simulink library "libbha_kinematic"  (R2015b)
settings: Solver=FixedStepDiscrete  StartTime=0.0  StopTime=Inf  FixedStep=0.004  RelTol=1e-3
PostLoadFcn:
  | , if any(exist('dsrtsu_mdlpostloadfcn', 'file') == [2, 3, 6]), try dsrtsu_mdlpostloadfcn('Execute', bdroot); catch fprintf('Error in PostLoadFcn (dsrtsu_mdlpostloadfcn) for model "%s":\n %s\n', bdroot, lasterr); end, end,
undefined symbols (not defined in the file or in its folder): BHA, BHASIM
libraries: libbha_kinematic x14
(part 3 of 3)

== matlab function libbha_kinematic/BHA_Kin_DirDiff_2ndO_CC_cont/J_general & J_specific ==
  data: h output; k output; q input; dot_q input; H_1b_w input; J_allg_kK output; r_i input; h_ih input; h_ib input; J_spez_kK_kA output; dot_J_allg_kK output; dot_J_spez_kK_kA output
function [h, k, J_allg_kK, J_spez_kK_kA, dot_J_allg_kK, dot_J_spez_kK_kA]   = Jacobi_CC_continuum(q, dot_q, H_1b_w, r_i, h_ih, h_ib)
n = 3;
% XXXXXXXXXXXXXXXXXXXXXXXXXXXXXXXXXXXXXXXXXXXXXXXXXXXXXXXXXXXXXXXXXXXXXXXXX
% Analytische Berechnung der Jacobi-Matrizen J_general und J_specific 
% - Modell - Constant Curvature Continuum
%
% Ansatz:
% h     = f_general(k)
% k     = f_specific(q)
% ==>
% h     = f_general(f_specific(q))
%
% J_general     = dh / dk
% J_specific    = dk / dq
%
% mit:
% q     = [ell_11, ell_12, ell_13, ell_21, ell_22, ell_23, ell_31, ell_32, ell_33]
% k     = [phi_1, kappa_1, ell_1, phi_2, kappa_2, ell_2, phi_3, kappa_3, ell_3]
% h     = [ H_1,1,  H_2,1,  H_3,1,  H_1,2,  H_2,2,  H_3,2,  H_1,3,  H_2,3,  H_3,3,  H_1,4,  H_2,4,  H_3,4]
%           1       2       3       4       5       6       7       8       9       10      11      12   
%
% Input:
%   q           [3nx1]  Zustandsvektor der Gelenkkoordinaten (Bogenlänge der Aktoren)
%   H_1b_w   [4x4]   Homogene Transformation: Koordinatensystem 1b
%                       relativ zum Weltsystem
%
% Output:
%   h           [12x1]  Pose des TCP (Homohene Transformation in Vektor geschrieben, ohne Zeile 0,0,0,1)
%   J_general   [12x3n] Allgemeingültige Jacobi-Matrix für kontinuierliche Manipulatoren
%   k           [3nx1]  Konfigurationszustand
%   J_specific  [3nx3n] Manipulator-spezifische Jacobimatrix (3-Aktuator Kontinuum Manipulator)
%
% Parameter:
%   n           [1x1]   Anzahl der Sektionen
%   r_i         [1xn]   Radialer Abstand der Aktoren pro Sektion
%   h_ib        [1xn]   Höhe der Sektionsbasis pro Sektion
%   h_ih        [1xn]   Höhe des Sektionskopfs pro Sektion
%
% Stand: 21.01.2013     Tobias Mahl
% XXXXXXXXXXXXXXXXXXXXXXXXXXXXXXXXXXXXXXXXXXXXXXXXXXXXXXXXXXXXXXXXXXXXXXXXX
    
    eps_kappa_i = 1e-7*ones(1, n);
    eps_wurzel_i= 1e-6*ones(1, n);% Berechnen!
    
    % Direkte Kinematik
    k = f_spez_kK_kA(n, q, r_i);
    [H_nh_w, H_ih_ib] = f_allg_kK(n, k, h_ib, h_ih, H_1b_w, eps_kappa_i);
    h = H2h(H_nh_w);
    
    % Direkte differentielle Kinematik 1. Ordnung
    J_spez_kK_kA = df_spez_kK_kA_dq(n, q, r_i, k, eps_wurzel_i);
    [J_allg_kK, dh_Ih_Ib_dk_I_all] = df_allg_kK_dk(n, k, h_ib, h_ih, H_1b_w, H_ih_ib, eps_kappa_i);
    
    % Direkte differentielle Kinematik 2. Ordnung
    dot_J_spez_kK_kA = dot_dk_dq(n, q, dot_q, r_i);
    
    ddH_nh_w_dk_dk = clc_ddH_nh_w_dk_dk(n, k, H_1b_w, H_ih_ib, dh_Ih_Ib_dk_I_all, h_ib, h_ih);
    dot_k = J_spez_kK_kA * dot_q;
    dot_J_allg_kK = ddf_allg_kK_dk_dt(n, dot_k, ddH_nh_w_dk_dk);
end

%% XXXXXXXXXXXXXXXXXXXXXXXXXXXXXX Allgemeines XXXXXXXXXXXXXXXXXXXXXXXXXXXXX

function h = H2h(H)
% Transformation:
%   homogene Transformation H --> vektorielle Repräsentation h
%                     H {4x4} --> h {12x1}

    h = reshape(H(1:3,:), [12,1]);
end

function H = h2H(h)
% Transformation:
%   vektorielle Repräsentation h --> homogene Transformation H
%                       h {12x1} --> H {4x4}

    H = [reshape(h, [3,4]); 0,0,0,1];
end

%% XXXXXXXXXXXXXXXXXXXXXXXXXXXXXX f_spez XXXXXXXXXXXXXXXXXXXXXXXXXXXXXXXXXX
function k = f_spez_kK_kA(n, q, r_i)
% Berechnung der Transformation
% Aktorbogenlängen q --> Konfigurationszustand k  
% des kontinuierlichen Roboters gemäß der Abbildung:
% k = f_specific(q)
% 
% Input:
%   q  [3nx1]   Aktorbogenlängen (kontinuierlich biegender Aktor)
%
% Output:
%   k     [3nx1]   Konfigurationszustand mit (phi_i, kappa_i, ell_i)
%
% Parameter:
%   r_i     [1xn]   Radiale Abständ der Aktoren je Sektion i
    
    k = zeros(3*n, 1);
    for ii=1:n
        k((1:3)+(ii-1)*3, 1) = f_spez_kK_kA_I(q((1:3)+(ii-1)*3, 1), r_i(ii));
    end
end

function k_I = f_spez_kK_kA_I(q_I, r_I)
% Berechnung der Transformation
% Aktorbogenlängen q_I --> Konfigurationszustand [phi_I, kappa_I, ell_I]  
% einer einzelnen Sektion gemäß der Abbildung:
% k_I = f_specific_I(q_I)
% 
% Input:
%   q_I  [3x1]   Aktorbogenlängen (kontinuierlich biegender Aktor)
%
% Output:
%   k_I     [3x1]   Konfigurationszustand (phi_I, kappa_I, ell_I)
%
% Parameter:
%   r_I     [1x1]   Radialer Abstand der Aktoren

    wurzel = sqrt(max([0, q_I(1,1)^2 + q_I(2,1)^2 + q_I(3,1)^2 - q_I(1,1)*q_I(2,1) - q_I(1,1)*q_I(3,1) - q_I(2,1)*q_I(3,1)]));
    
    phi_I  = atan2(sqrt(3)*(q_I(3,1)-q_I(2,1)), q_I(2,1)+q_I(3,1)-2*q_I(1,1));
    kappa_I= 2*wurzel / (r_I*(q_I(1,1)+q_I(2,1)+q_I(3,1)));
    ell_I  = (q_I(1,1)+q_I(2,1)+q_I(3,1))/3;
    
    k_I    = [phi_I; kappa_I; ell_I];
end

%% XXXXXXXXXXXXXXXXXXXXXXXXXXXXXX f_allg XXXXXXXXXXXXXXXXXXXXXXXXXXXXXXXXXX
function [H_nh_w, H_ih_ib] = f_allg_kK(n, k, h_ib, h_ih, H_1b_w, eps_kappa_i)
% Berechnung der homogenen Transformation der I-ten Sektion gemäß Abbildung
% H = f_general_H(k, h_ib, h_ih, H_1b_w)
% 
% Input:
%   k           Konfigurationszustand (phi_i, kappa_i, ell_i) aller Sektionen
%   h_ib        Höhen der Sektionsfüsse (Sektionen i)
%   h_ih        Höhen des Sektionsköpfe (Sektionen i)
%   eps_kappa_i Minimale Krümmung für die ungleich Gerade gerechnet wird (Sektionen i)
%
% Output:   
%   H_nh_w  Homogene Transformation zwischen n-tem Kopf- und Welt-Koordinatensystem

    H_nh_w  = H_1b_w;
    H_ih_ib = zeros(4, 4, n);
    
    for ii = 1:n
        H_Ih_Ib         = f_allg_kK_I(k((1:3)+(ii-1)*3, 1), h_ib(ii), h_ih(ii), eps_kappa_i(ii));
        H_nh_w          = H_nh_w*H_Ih_Ib;
        H_ih_ib(:,:,ii) = H_Ih_Ib;
    end
end

function H_Ih_Ib = f_allg_kK_I(k_I, h_Ib, h_Ih, eps_kappa_I)
% Berechnung der homogenen Transformation der I-ten Sektion gemäß Abbildung
% H_I = f_general_H_I(k_I, h_Ib, h_Ih)
% 
% Input:
%   k           Konfigurationszustand (phi_I, kappa_I, ell_I) der Sektion I
%   h_Ib        Höhe der Sektionsbasis (Sektion I)
%   h_Ih        Höhe des Sektionskopfs (Sektion I)
%   eps_kappa_I Minimale Krümmung für die ungleich Gerade gerechnet wird (Sektione I)
%
% Output:   
%   H_Ih_Ib Homogene Transformation zwischen Kopf- und Basis-Koordinatensystem

    % homogene Transformation der Basis
    H_I0_Ib = [eye(3), [0; 0; h_Ib];...
               0,0,0,  1];

    % homogene Transformation des Kopfs
    H_Ih_I1 = [eye(3), [0; 0; h_Ih];...
               0,0,0,  1];

    % homogene Transformation des Aktorbereichs
    % Berechnung gemäß lim kappa->0 (Biegelinie ist eine Gerade)
    if(k_I(2) < eps_kappa_I)
        R_I1_I0 = eye(3);
        o_I1_I0 = [0; 0; k_I(3)];

    % Berechnung gemäß kappa>0 (Biegelinie ist ein Kreissegment)
    else
        s_phi   = sin(k_I(1));
        c_phi   = cos(k_I(1));
        s_kl    = sin(k_I(2)*k_I(3));
        c_kl    = cos(k_I(2)*k_I(3));

        R_I1_I0 = [c_phi^2*(c_kl-1)+1,      s_phi*c_phi*(c_kl-1),       c_phi*s_kl;...
                   s_phi*c_phi*(c_kl-1),    c_phi^2*(1-c_kl)+c_kl,      s_phi*s_kl;...
                   -c_phi*s_kl,             -s_phi*s_kl,                c_kl];

        o_I1_I0 = [c_phi*(1-c_kl)/k_I(2);...
                   s_phi*(1-c_kl)/k_I(2);...
                   s_kl/k_I(2)];
    end
    H_I1_I0 = [R_I1_I0, o_I1_I0;...
               0,0,0,   1];

    H_Ih_Ib = H_I0_Ib*H_I1_I0*H_Ih_I1;
end

%% XXXXXXXXXXXXXXXXXXXXXXX J_spez XXXXXXXXXXXXXXXXXXXXXXXXXXXXXXXXXXXXXXXXX
function [J_spez_kK_kA] = df_spez_kK_kA_dq(n, q, r_i, k, eps_wurzel_i)
% Jakobimatrix der Trafo: Actuator space --> Configuration Space
% dk/dq  = J_specific(q)
% mit:
% k     = [phi_1, kappa_1, ell_1, phi_2, kappa_2, ell_2, phi_3, kappa_3, ell_3]
% q     = [ell_11, ell_12, ell_13, ell_21, ell_22, ell_23, ell_31, ell_32, ell_33]

    J_spez_kK_kA    = zeros(3*n, 3*n);
    for ii = 1:n
        q_I             = q((1:3)+3*(ii-1), 1);
        r_I             = r_i(ii);
        eps_wurzel_I    = eps_wurzel_i(ii);        

        % Singularität für wurzel=0 ! -> Definition des singulären Gebiets
        wurzel  = sqrt(max([0, q_I(1,1)^2 + q_I(2,1)^2 + q_I(3,1)^2 - q_I(1,1)*q_I(2,1) - q_I(1,1)*q_I(3,1) - q_I(2,1)*q_I(3,1)]));

        % Regularisierung der Singularität
        if wurzel < eps_wurzel_I
            %disp(['Regularisierung: wurzel = ', num2str(wurzel), ' < ', num2str(eps)])

            q_mean     = (q_I(1,1)+q_I(2,1)+q_I(3,1))/3;
            q_I(1,1)   = q_mean-eps_wurzel_I;
            q_I(2,1)   = q_mean;
            q_I(3,1)   = q_mean+eps_wurzel_I;
    
            k((1:3)+3*(ii-1), 1) = f_spez_kK_kA_I(q_I, r_I);
        end
        
        J_spez_kK_kA((1:3)+3*(ii-1), (1:3)+3*(ii-1)) = df_spez_kK_kA_dq_I(q_I, r_I);
    end
end

function J_spez_kK_kA_I = df_spez_kK_kA_dq_I(q_I, r_I)
% Berechnung der Jacobimatrix der Transformation
% Aktorbogenlängen q_I --> Konfigurationszustand [phi_I, kappa_I, ell_I]  
% einer einzelnen Sektion gemäß der Abbildung:
% dk_I / dq_I = df_spez_kK_kA_dq_I(q_I)
% 
% Input:
%   q_I  [3x1]   Aktorbogenlängen (kontinuierlich biegender Aktor)
%
% Output:
%   df_spez_kK_kA_dq_I    [3x3]   Jacobimatrix einer Sektion
%
% Parameter:
%   r_I     [1x1]   Radialer Abstand der Aktoren
    
    ell_sum= (q_I(1,1)+q_I(2,1)+q_I(3,1));
    wurzel = sqrt(max([0, q_I(1,1)^2 + q_I(2,1)^2 + q_I(3,1)^2 - q_I(1,1)*q_I(2,1) - q_I(1,1)*q_I(3,1) - q_I(2,1)*q_I(3,1)]));
    
    d_phi_dell1     =  sqrt(3)/2*(q_I(3,1)-q_I(2,1)) / wurzel^2;
    d_phi_dell2     = -sqrt(3)/2*(q_I(3,1)-q_I(1,1)) / wurzel^2;
    d_phi_dell3     =  sqrt(3)/2*(q_I(2,1)-q_I(1,1)) / wurzel^2;
    
    d_kappa_dell1   = 3*(q_I(1,1)*q_I(2,1) + q_I(1,1)*q_I(3,1) - q_I(2,1)^2 - q_I(3,1)^2) / (wurzel*r_I*ell_sum^2);
    d_kappa_dell2   = 3*(q_I(1,1)*q_I(2,1) + q_I(2,1)*q_I(3,1) - q_I(1,1)^2 - q_I(3,1)^2) / (wurzel*r_I*ell_sum^2);
    d_kappa_dell3   = 3*(q_I(1,1)*q_I(3,1) + q_I(2,1)*q_I(3,1) - q_I(1,1)^2 - q_I(2,1)^2) / (wurzel*r_I*ell_sum^2);

    d_ell_dell1     = 1/3;
    d_ell_dell2     = 1/3;
    d_ell_dell3     = 1/3;
    
    
    J_spez_kK_kA_I  = [d_phi_dell1,    d_phi_dell2,    d_phi_dell3;
                       d_kappa_dell1,  d_kappa_dell2,  d_kappa_dell3
                       d_ell_dell1,    d_ell_dell2,    d_ell_dell3   ];
end

%% XXXXXXXXXXXXXXXXXXXXXXX dot_J_spez XXXXXXXXXXXXXXXXXXXXXXXXXXXXXXXXXXXXX
function dot_J_spez_kK_kA = dot_dk_dq(n, q, dot_q, r_i)

    dot_J_spez_kK_kA = zeros(3*n, 3*n);
    for ii = 1:n
        q_I     = q((1:3)+3*(ii-1), 1);
        dot_q_I = dot_q((1:3)+3*(ii-1), 1);
        r_I     = r_i(ii);
        
        dot_J_spez_kK_kA((1:3)+3*(ii-1), (1:3)+3*(ii-1)) = dot_J_spez_kK_kA_I(q_I, dot_q_I, r_I);
    end
end

function dot_dk_I_dq_I = dot_J_spez_kK_kA_I(q_I, dot_q_I, r_I)

    dot_dk_I_dq_I = zeros(3,3);
    
    ddk_I_dq_I_dq_I = ddf_spez_kK_kA_I_dq_I_dq_I(q_I, r_I);
    for xi = 1:3
        for k = 1:3
            for chi = 1:3
                dot_dk_I_dq_I(xi, k) = dot_dk_I_dq_I(xi, k) + ddk_I_dq_I_dq_I(k, chi, xi)*dot_q_I(chi);
            end
        end
    end
end

% KKKKK Partielle Ableitung 2.Ord ddf_spez_kK_kA_I_dq_Ik_dq_Ixi KKKKKKKKKKK
function ddk_I_dq_I_dq_I = ddf_spez_kK_kA_I_dq_I_dq_I(q_I, r_I)
% Input:
%   - q_I = [ell_i1, ell_i2, ell_i3]^T       Aktorzustand
%   - r_I                                    Seilzugabstand
%
% Output:
%   - ddk_I_dq_I_dq_I   [dim_q_I x dim_q_I x dim_k_I]   Partielle Ableitung 2.Ord. von allen Konfigurationszuständen k_I nach allen Aktorzuständen q_I 
 
    ddk_I_dq_I_dq_I = zeros(3,3,3);
    
    q1 = q_I(1);
    q2 = q_I(2);
    q3 = q_I(3);
    
    % Vermeidung Singularität
    q_dist_eps  = 1e-15;
    q_dist      = q1 ^ 2 + q2 ^ 2 + q3 ^ 2 - q1 * q2 - q1 * q3 - q2 * q3;
    while (q_dist<q_dist_eps)
        q1      = q1-5e-8;
        q_dist  = q1 ^ 2 + q2 ^ 2 + q3 ^ 2 - q1 * q2 - q1 * q3 - q2 * q3;
    end

    % Substitutionen
    q_sum   = q1 + q2 + q3;

    % Ableitungen / Hesse-matrizen
    d2ka_dqbdqc = zeros(3*3, 3);
    
    % d2k1_dqbdqc
    mddphi_dq1dq1 = -sqrt(0.3e1) * (q3 - q2) / q_dist ^ 2 * (-q2 - q3 + 2 * q1) / 0.2e1;
    mddphi_dq1dq2 = -sqrt(0.3e1) * (-q2 ^ 2 + 2 * q2 * q3 - 2 * q3 * q1 + q1 ^ 2) / q_dist ^ 2 / 0.2e1;
    mddphi_dq1dq3 = sqrt(0.3e1) * (2 * q2 * q3 - 2 * q2 * q1 - q3 ^ 2 + q1 ^ 2) / q_dist ^ 2 / 0.2e1;
    
    mddphi_dq2dq1 = mddphi_dq1dq2;
    mddphi_dq2dq2 = sqrt(0.3e1) * (-q3 + q1) * (-2 * q2 + q3 + q1) / q_dist ^ 2 / 0.2e1;
    mddphi_dq2dq3 = -sqrt(0.3e1) * (q2 ^ 2 - 2 * q2 * q1 - q3 ^ 2 + 2 * q3 * q1) / q_dist ^ 2 / 0.2e1;
    
    mddphi_dq3dq1 = mddphi_dq1dq3;
    mddphi_dq3dq2 = mddphi_dq2dq3;
    mddphi_dq3dq3 = -sqrt(0.3e1) * (-q2 + q1) * (q2 - 2 * q3 + q1) / q_dist ^ 2 / 0.2e1;
    
    ddk_I_dq_I_dq_I(:,:, 1) = [ mddphi_dq1dq1, mddphi_dq2dq1, mddphi_dq3dq1;
                                mddphi_dq1dq2, mddphi_dq2dq2, mddphi_dq3dq2;
                                mddphi_dq1dq3, mddphi_dq2dq3, mddphi_dq3dq3];
    
    % dk2_dqbdqc
    mddkappa_dq1dq1 = -0.3e1 / 0.2e1 * (-6 * q2 * q1 ^ 2 * q3 + 6 * q2 * q1 * q3 ^ 2 + 6 * q2 ^ 2 * q1 * q3 - 9 * q2 ^ 2 * q1 ^ 2 - 5 * q2 ^ 4 - 5 * q3 ^ 4 + 4 * q3 ^ 3 * q2 + 6 * q2 ^ 3 * q1 + 4 * q2 * q1 ^ 3 + 4 * q2 ^ 3 * q3 - 6 * q2 ^ 2 * q3 ^ 2 - 9 * q3 ^ 2 * q1 ^ 2 + 6 * q3 ^ 3 * q1 + 4 * q3 * q1 ^ 3) * (q_dist ^ (-0.3e1 / 0.2e1)) / r_I / (q_sum ^ 3);
    mddkappa_dq1dq2 = 0.3e1 / 0.2e1 * (2 * q2 ^ 4 + 3 * q3 ^ 4 + 3 * q2 * q1 ^ 2 * q3 + 3 * q2 ^ 2 * q1 * q3 - 3 * q2 * q1 * q3 ^ 2 + 6 * q2 ^ 2 * q1 ^ 2 - 7 * q2 ^ 3 * q1 - 7 * q2 * q1 ^ 3 - 3 * q2 ^ 3 * q3 + 9 * q2 ^ 2 * q3 ^ 2 - 3 * q3 * q1 ^ 3 + 9 * q3 ^ 2 * q1 ^ 2 - 7 * q3 ^ 3 * q2 - 7 * q3 ^ 3 * q1 + 2 * q1 ^ 4) * (q_dist ^ (-0.3e1 / 0.2e1)) / r_I / (q_sum ^ 3);
    mddkappa_dq1dq3 = 0.3e1 / 0.2e1 * (3 * q2 ^ 4 + 2 * q3 ^ 4 + 3 * q2 * q1 ^ 2 * q3 - 3 * q2 ^ 2 * q1 * q3 + 3 * q2 * q1 * q3 ^ 2 + 9 * q2 ^ 2 * q1 ^ 2 - 7 * q2 ^ 3 * q1 - 3 * q2 * q1 ^ 3 - 7 * q2 ^ 3 * q3 + 9 * q2 ^ 2 * q3 ^ 2 - 7 * q3 * q1 ^ 3 + 6 * q3 ^ 2 * q1 ^ 2 - 3 * q3 ^ 3 * q2 - 7 * q3 ^ 3 * q1 + 2 * q1 ^ 4) * (q_dist ^ (-0.3e1 / 0.2e1)) / r_I / (q_sum ^ 3);
    
    mddkappa_dq2dq1 = mddkappa_dq1dq2;
    mddkappa_dq2dq2 = 0.3e1 / 0.2e1 * (5 * q3 ^ 4 - 6 * q2 * q1 ^ 2 * q3 + 6 * q2 ^ 2 * q1 * q3 - 6 * q2 * q1 * q3 ^ 2 + 9 * q2 ^ 2 * q1 ^ 2 - 4 * q2 ^ 3 * q1 - 6 * q2 * q1 ^ 3 - 4 * q2 ^ 3 * q3 + 9 * q2 ^ 2 * q3 ^ 2 - 4 * q3 * q1 ^ 3 + 6 * q3 ^ 2 * q1 ^ 2 - 6 * q3 ^ 3 * q2 - 4 * q3 ^ 3 * q1 + 5 * q1 ^ 4) * (q_dist ^ (-0.3e1 / 0.2e1)) / r_I / (q_sum ^ 3);
    mddkappa_dq2dq3 = 0.3e1 / 0.2e1 * (2 * q2 ^ 4 + 2 * q3 ^ 4 - 3 * q2 * q1 ^ 2 * q3 + 3 * q2 ^ 2 * q1 * q3 + 3 * q2 * q1 * q3 ^ 2 + 9 * q2 ^ 2 * q1 ^ 2 - 3 * q2 ^ 3 * q1 - 7 * q2 ^ 3 * q3 + 6 * q2 ^ 2 * q3 ^ 2 - 7 * q2 * q3 ^ 3 - 3 * q3 ^ 3 * q1 + 9 * q3 ^ 2 * q1 ^ 2 - 7 * q1 ^ 3 * q3 - 7 * q1 ^ 3 * q2 + 3 * q1 ^ 4) * (q_dist ^ (-0.3e1 / 0.2e1)) / r_I / (q_sum ^ 3);

    mddkappa_dq3dq1 = mddkappa_dq1dq3;
    mddkappa_dq3dq2 = mddkappa_dq2dq3;
    mddkappa_dq3dq3 = 0.3e1 / 0.2e1 * (5 * q2 ^ 4 - 6 * q2 * q1 ^ 2 * q3 - 6 * q2 ^ 2 * q1 * q3 + 6 * q2 * q1 * q3 ^ 2 + 6 * q2 ^ 2 * q1 ^ 2 - 4 * q2 ^ 3 * q1 - 6 * q2 ^ 3 * q3 + 9 * q2 ^ 2 * q3 ^ 2 - 4 * q2 * q3 ^ 3 - 4 * q3 ^ 3 * q1 + 9 * q3 ^ 2 * q1 ^ 2 - 6 * q1 ^ 3 * q3 - 4 * q1 ^ 3 * q2 + 5 * q1 ^ 4) * (q_dist ^ (-0.3e1 / 0.2e1)) / r_I / (q_sum ^ 3);

    ddk_I_dq_I_dq_I(:,:, 2) = [ mddkappa_dq1dq1, mddkappa_dq2dq1, mddkappa_dq3dq1;
                                mddkappa_dq1dq2, mddkappa_dq2dq2, mddkappa_dq3dq2;
                                mddkappa_dq1dq3, mddkappa_dq2dq3, mddkappa_dq3dq3];
    
    % dk3_dqbdqc
    % partielle Ableitungen 2. Ord von ell sind alle 0
end


%% XXXXXXXXXXXXXXXXXXXXXXX J_allg XXXXXXXXXXXXXXXXXXXXXXXXXXXXXXXXXXXXXXXXX
function [J_allg_kK, dh_Ih_Ib_dk_I_all]  = df_allg_kK_dk(n, k, h_ib, h_ih, H_1b_w, H_ih_ib, eps_kappa_i)
% Funktion zur Berechnung der Jacobimatrix eines Continuum Manipulators
%
% Trafo: Configuration Space --> Task Space
% h = f_general(k)
%
% h     = [ H_1,1,  H_2,1,  H_3,1,  H_1,2,  H_2,2,  H_3,2,  H_1,3,  H_2,3,  H_3,3,  H_1,4,  H_2,4,  H_3,4]
%           1       2       3       4       5       6       7       8       9       10      11      12   
% k     = [phi_1, kappa_1, ell_1, phi_2, kappa_2, ell_2, phi_3, kappa_3, ell_3]
%

    J_allg_kK           = zeros(12, 3*n);
    dh_Ih_Ib_dk_I_all   = zeros(12, 3*n); % = [df_allg_kK_1_dk_11 ... df_allg_kK_n_dk_n3]
    for ii = 1:n
        % Ableitungstensor der I-ten Sektion
        dH_Ih_Ib_dk_I = df_allg_kK_dk_I(k((1:3)+3*(ii-1), 1), h_ib(ii), h_ih(ii), eps_kappa_i(ii));
        dh_Ih_Ib_dk_I_all(:, (1:3)+3*(ii-1)) = [H2h(dH_Ih_Ib_dk_I(:,:,1)),...
                                                H2h(dH_Ih_Ib_dk_I(:,:,2)),...
                                                H2h(dH_Ih_Ib_dk_I(:,:,3))];
        
        % Ableitungstensor des TCP nach den Konfigurationsparametern der I-ten Sektion 
        dH_nh_w_dk_I = zeros(4,4,3);
        
        % Ableitungsregel dH/dk_IJ = H_1b_w * H_I-1h_in_1b * dH_Ih_in_Ib/dk_IJ * H_nh_in_I+1b 
        H_Imh_1b = eye(4);
        for xi = 1:ii-1
            H_Imh_1b = H_Imh_1b*H_ih_ib(:,:,xi);
        end
        H_nh_Ipb = eye(4);
        for xi = ii+1:n
            H_nh_Ipb = H_nh_Ipb*H_ih_ib(:,:,xi);
        end
        
        dH_nh_w_dk_I(:,:,1) = H_1b_w*H_Imh_1b* dH_Ih_Ib_dk_I(:,:,1) *H_nh_Ipb;
        dH_nh_w_dk_I(:,:,2) = H_1b_w*H_Imh_1b* dH_Ih_Ib_dk_I(:,:,2) *H_nh_Ipb;
        dH_nh_w_dk_I(:,:,3) = H_1b_w*H_Imh_1b* dH_Ih_Ib_dk_I(:,:,3) *H_nh_Ipb;
        
        % Jacobimatrix
        J_allg_kK(:, (1:3)+3*(ii-1)) = [H2h(dH_nh_w_dk_I(:,:,1)),...
                                        H2h(dH_nh_w_dk_I(:,:,2)),...
                                        H2h(dH_nh_w_dk_I(:,:,3))];
    end
end

function dH_Ih_Ib_dk_I = df_allg_kK_dk_I(k_I, h_Ib, h_Ih, eps_kappa_I)
% Berechnung des Ableitungstensors der homogenen Transformation der I-ten Sektion S_Ih_in_Ib
% 
% Input:
%   k           Konfigurationszustand (phi_I, kappa_I, ell_I) der Sektion I
%   h_Ib        Höhe der Sektionsbasis (Sektion I)
%   h_Ih        Höhe des Sektionskopfs (Sektion I)
%   eps_kappa_I Minimale Krümmung für die ungleich Gerade gerechnet wird (Sektione I)
%
% Output:   
%   dH_Ih_Ib_dk_I   Ableitungstensor [4x4x3] der homogenen Transformation zwischen Kopf- und Fuß-Koordinatensystem

    %% homogene Transformation des Fußes
    H_I0_Ib = [eye(3), [0; 0; h_Ib];...
               0,0,0,  1];

    %% homogene Transformation des Kopfs
    H_Ih_I1 = [eye(3), [0; 0; h_Ih];...
               0,0,0,  1];
           
    %% homogene Transformation des Aktorbereichs
    % Ableitungstensor
    dH_Ih_Ib_dk_I = zeros(4,4,3);

    % Berechnung gemäß lim kappa->0 (Biegelinie ist eine Gerade)
    if(k_I(2) < eps_kappa_I)
        dH_Ih_Ib_dk_I(3,4,3) = 1;

    % Berechnung gemäß kappa>0 (Biegelinie ist ein Kreissegment)
    else
        s_phi   = sin(k_I(1));
        c_phi   = cos(k_I(1));
        s_kl    = sin(k_I(2)*k_I(3));
        c_kl    = cos(k_I(2)*k_I(3));

        % Ableitung der Homogenen Trafo nach dphi_I
        d_H_I1_I0_dphi   = [-2*s_phi*c_phi*(c_kl-1),            c_phi^2*(c_kl-1)-s_phi^2*(c_kl-1),  -s_phi*s_kl,    -s_phi*(1-c_kl)/k_I(2);
                            c_phi^2*(c_kl-1)-s_phi^2*(c_kl-1),  -2*c_phi*(1-c_kl)*s_phi,            c_phi*s_kl,     c_phi*(1-c_kl)/k_I(2);
                            s_phi*s_kl,                         -c_phi*s_kl,                        0,              0;
                            0,                                  0,                                  0,              0                           ];

        dH_Ih_Ib_dk_I(:,:,1) = H_I0_Ib * d_H_I1_I0_dphi * H_Ih_I1;

        % Ableitung der Homogenen Trafo nach dkappa_I
        d_H_I1_I0_dkappa = [-c_phi^2*s_kl*k_I(3),            -s_phi*c_phi*s_kl*k_I(3),                c_phi*c_kl*k_I(3),   c_phi*s_kl*k_I(3)/k_I(2) - c_phi*(1-c_kl)/k_I(2)^2;
                            -s_phi*c_phi*s_kl*k_I(3),        c_phi^2*s_kl*k_I(3) - s_kl*k_I(3),       s_phi*c_kl*k_I(3),   s_phi*s_kl*k_I(3)/k_I(2) - s_phi*(1-c_kl)/k_I(2)^2;
                            -c_phi*c_kl*k_I(3),              -s_phi*c_kl*k_I(3),                      -s_kl*k_I(3),        c_kl*k_I(3)/k_I(2) - s_kl/k_I(2)^2;
                            0,                               0,                                       0,                   0                                                   ];

        dH_Ih_Ib_dk_I(:,:,2) = H_I0_Ib * d_H_I1_I0_dkappa * H_Ih_I1;
        
        % Ableitung der Homogenen Trafo nach dell_I
        d_H_I1_I0_dell   = [-c_phi^2*s_kl*k_I(2),          -s_phi*c_phi*s_kl*k_I(2),              c_phi*c_kl*k_I(2), c_phi*s_kl;
                            -s_phi*c_phi*s_kl*k_I(2),      c_phi^2*s_kl*k_I(2) - s_kl*k_I(2),     s_phi*c_kl*k_I(2), s_phi*s_kl;
                            -c_phi*c_kl*k_I(2),            -s_phi*c_kl*k_I(2),                    -s_kl*k_I(2),      c_kl;
                            0,                              0,                                      0,                  0           ];
            
        dH_Ih_Ib_dk_I(:,:,3) = H_I0_Ib * d_H_I1_I0_dell * H_Ih_I1;
    end
end

%% XXXXXXXXXXXXXXXXXXXXXXX dot_J_allg XXXXXXXXXXXXXXXXXXXXXXXXXXXXXXXXXXXXX
function [dot_J_allg_kK] = ddf_allg_kK_dk_dt(n, dot_k, ddH_nh_w_dk_dk)
% 
%     dot_J_allg_kK   = zeros(12, 3*n);
%     
    
    dot_J_allg_kK = zeros(12, 3*n);
    for xi = 1:3*n
        for chi = 1:3*n
            dot_J_allg_kK(:, chi) = H2h( ddH_nh_w_dk_dk((1:4)+4*(xi-1), (1:4)+4*(chi-1)).*dot_k(xi) );
        end
    end
end

% HHHHHHHHHHHHH Partielle Ableitung 2.Ord nach ki HHHHHHHHHHHHHHHHHHHHHHHH
function [ddH_nh_w_dk_dk] = clc_ddH_nh_w_dk_dk(n, k, H_1b_w, H_ih_ib, dh_Ih_Ib_dk_I_all, h_ib, h_ih)
% Input:
%   - k_I = [phi, kappa, ell]^T     Konfigurationszustand
%   - h_ib                          Höhe der Sektionsbasis (alle Sektionen)
%   - h_ih                          Höhe des Sektionskopfs (alle Sektionen)
%
% Output
%   - ddH_nh_w_dk_dk   [4*dim_k x 4*dim_k]       Partielle Ableitung 2.Ord von H_nh_w nach allen Konfigurationszuständen k_I 
    
    ddH_nh_w_dk_dk = zeros(4*3*n, 4*3*n);
    for xi = 1:n
        for ii = 1:xi
            if ii==xi
                H_imh_w = H_1b_w;
                for nn = 1:ii-1
                    H_imh_w = H_imh_w * H_ih_ib(:,:,nn);
                end
                H_ximh_ipb = eye(4);
                for nn = ii+1:xi-1
                    H_ximh_ipb = H_ximh_ipb * H_ih_ib(:,:,nn);
                end
                H_nh_xipb = eye(4);
                for nn = xi+1:n
                    H_nh_xipb = H_nh_xipb * H_ih_ib(:,:,nn);
                end
                for nu = 1:3
                    for chi = 1:3
                        dH_Ih_Ib_dk_ik      = h2H(dh_Ih_Ib_dk_I_all(:, 3*(ii-1)+nu));
                        dH_Ih_Ib_dk_xichi   = h2H(dh_Ih_Ib_dk_I_all(:, 3*(xi-1)+chi));
                        ddH_nh_w_dk_dk((1:4)+4*(chi-1)+(xi-1)*3*4, (1:4)+4*(nu-1)+(ii-1)*3*4) =...
                            H_imh_w * dH_Ih_Ib_dk_ik *H_ximh_ipb* dH_Ih_Ib_dk_xichi *H_nh_xipb;
                        ddH_nh_w_dk_dk((1:4)+4*(nu-1)+(ii-1)*3*4, (1:4)+4*(chi-1)+(xi-1)*3*4) =...
                            ddH_nh_w_dk_dk((1:4)+4*(chi-1)+(xi-1)*3*4, (1:4)+4*(nu-1)+(ii-1)*3*4);
                    end
                end
            else
                H_imh_w = H_1b_w;
                for nn = 1:ii-1
                    H_imh_w = H_imh_w * H_ih_ib(:,:,nn);
                end
                H_nh_ipb = eye(4);
                for nn = ii+1:n
                    H_nh_ipb = H_nh_ipb * H_ih_ib(:,:,nn);
                end
                ddH_Ih_Ib_dk_I_dk_I = clc_ddH_Ih_Ib_dk_I_dk_I(k((1:3)+3*(ii-1)), h_ib(ii), h_ih(ii));
                ddH_nh_w_dk_dk((1:3*4)+(xi-1)*3*4, (1:3*4)+(ii-1)*3*4) = ...
                    clc_Trafo_H( clc_Trafo_H(H_imh_w, ddH_Ih_Ib_dk_I_dk_I), H_nh_ipb);
            end
        end
    end
end


% HHHHHHHHHHHHH Partielle Ableitung 2.Ord nach ki HHHHHHHHHHHHHHHHHHHHHHHH
function [ddH_Ih_Ib_dk_I_dk_I] = clc_ddH_Ih_Ib_dk_I_dk_I(k_I, h_Ib, h_Ih)
% Input:
%   - k_I = [phi, kappa, ell]^T     Konfigurationszustand
%   - h_Ib                          Höhe der Sektionsbasis (Sektion I)
%   - h_Ih                          Höhe des Sektionskopfs (Sektion I)
%
% Output
%   - ddH_Ih_Ib_dk_I_dk_I   [4*dim_k_I x 4*dim_k_I]       Partielle Ableitung 2.Ord von H_Ih_Ib nach allen Konfigurationszuständen k_I 
    
    H_I0_Ib         = [eye(3), [0; 0; h_Ib]; 0, 0, 0, 1];
    H_Ih_I1         = [eye(3), [0; 0; h_Ih]; 0, 0, 0, 1];
    
    ddH_Ih_Ib_dk_I_dk_I = clc_Trafo_H( clc_Trafo_H(H_I0_Ib, clc_ddH_I1_I0_dk_I_dk_I(k_I)) , H_Ih_I1);
end

% HHHHHHHHHHHHH Partielle Ableitung 2.Ord nach ki HHHHHHHHHHHHHHHHHHHHHHHH
function [ddH_I1_I0_dk_I_dk_I] = clc_ddH_I1_I0_dk_I_dk_I(k_I)
% Input:
%   - k_I = [phi, kappa, ell]^T              Konfigurationszustand
%
% Output
%   - ddH_I1_I0_dk_I_dk_I   [4*dim_k_I x 4*dim_k_I]       Partielle Ableitung 2.Ord von H_I1_I0 nach allen Konfigurationszuständen k_I 
    
    k1 = k_I(1);
    k2 = k_I(2);
    k3 = k_I(3);

    % Vermeidung Singularität
    k2_eps = 1e-6;
    k2     = max([k2_eps, k2]);
    
    % Substitutionen
    sk1     = sin(k1);
    ck1     = cos(k1);
    sk2k3   = sin(k2 * k3);
    ck2k3   = cos(k2 * k3);
    
    dim_k_I = 3;
    ddH_I1_I0_dk_I_dk_I = zeros(4*dim_k_I, 4*dim_k_I);
    
% d2H_i_in_im1_dk1dk1
    mddH_i_in_im1_dk1dk1_11 = -0.4e1 * ck2k3 * ck1 ^ 2 + 0.2e1 * ck2k3 + 0.4e1 * ck1 ^ 2 - 0.2e1;
    mddH_i_in_im1_dk1dk1_12 = -0.4e1 * sk1 * ck1 * (ck2k3 - 0.1e1);
    mddH_i_in_im1_dk1dk1_13 = -ck1 * sk2k3;
    mddH_i_in_im1_dk1dk1_14 = ck1 * (ck2k3 - 0.1e1) / k2;
    
    mddH_i_in_im1_dk1dk1_21 = -0.4e1 * sk1 * ck1 * (ck2k3 - 0.1e1);
    mddH_i_in_im1_dk1dk1_22 = 0.4e1 * ck2k3 * ck1 ^ 2 - 0.2e1 * ck2k3 - 0.4e1 * ck1 ^ 2 + 0.2e1;
    mddH_i_in_im1_dk1dk1_23 = -sk1 * sk2k3;
    mddH_i_in_im1_dk1dk1_24 = sk1 * (ck2k3 - 0.1e1) / k2;
    
    mddH_i_in_im1_dk1dk1_31 = ck1 * sk2k3;
    mddH_i_in_im1_dk1dk1_32 = sk1 * sk2k3;
    mddH_i_in_im1_dk1dk1_33 = 0;
    mddH_i_in_im1_dk1dk1_34 = 0;
    
    ddH_I1_I0_dk_I_dk_I(1:3, 1:4)       = [mddH_i_in_im1_dk1dk1_11, mddH_i_in_im1_dk1dk1_12, mddH_i_in_im1_dk1dk1_13, mddH_i_in_im1_dk1dk1_14;
                                           mddH_i_in_im1_dk1dk1_21, mddH_i_in_im1_dk1dk1_22, mddH_i_in_im1_dk1dk1_23, mddH_i_in_im1_dk1dk1_24;
                                           mddH_i_in_im1_dk1dk1_31, mddH_i_in_im1_dk1dk1_32, mddH_i_in_im1_dk1dk1_33, mddH_i_in_im1_dk1dk1_34 ]; 
    
    
    % d2H_i_in_im1_dk2dk2
    mddH_i_in_im1_dk2dk2_11 = -ck1 ^ 2 * ck2k3 * k3 ^ 2;
    mddH_i_in_im1_dk2dk2_12 = -sk1 * ck1 * ck2k3 * k3 ^ 2;
    mddH_i_in_im1_dk2dk2_13 = -ck1 * sk2k3 * k3 ^ 2;
    mddH_i_in_im1_dk2dk2_14 = -ck1 * (-ck2k3 * k3 ^ 2 * k2 ^ 2 + 0.2e1 * sk2k3 * k3 * k2 + 0.2e1 * ck2k3 - 0.2e1) / k2 ^ 3;
    
    mddH_i_in_im1_dk2dk2_21 = -sk1 * ck1 * ck2k3 * k3 ^ 2;
    mddH_i_in_im1_dk2dk2_22 = -ck2k3 * k3 ^ 2 * sk1 ^ 2;
    mddH_i_in_im1_dk2dk2_23 = -sk1 * sk2k3 * k3 ^ 2;
    mddH_i_in_im1_dk2dk2_24 = -sk1 * (-ck2k3 * k3 ^ 2 * k2 ^ 2 + 0.2e1 * sk2k3 * k3 * k2 + 0.2e1 * ck2k3 - 0.2e1) / k2 ^ 3;
    
    mddH_i_in_im1_dk2dk2_31 = ck1 * sk2k3 * k3 ^ 2;
    mddH_i_in_im1_dk2dk2_32 = sk1 * sk2k3 * k3 ^ 2;
    mddH_i_in_im1_dk2dk2_33 = -ck2k3 * k3 ^ 2;
    mddH_i_in_im1_dk2dk2_34 = -(sk2k3 * k3 ^ 2 * k2 ^ 2 + 0.2e1 * ck2k3 * k3 * k2 - 0.2e1 * sk2k3) / k2 ^ 3;
    
    ddH_I1_I0_dk_I_dk_I(5:7, 5:8)       = [mddH_i_in_im1_dk2dk2_11, mddH_i_in_im1_dk2dk2_12, mddH_i_in_im1_dk2dk2_13, mddH_i_in_im1_dk2dk2_14;
                                           mddH_i_in_im1_dk2dk2_21, mddH_i_in_im1_dk2dk2_22, mddH_i_in_im1_dk2dk2_23, mddH_i_in_im1_dk2dk2_24;
                                           mddH_i_in_im1_dk2dk2_31, mddH_i_in_im1_dk2dk2_32, mddH_i_in_im1_dk2dk2_33, mddH_i_in_im1_dk2dk2_34 ]; 
                                       
    % d2H_i_in_im1_dk3dk3
    mddH_i_in_im1_dk3dk3_11 = -ck1 ^ 2 * ck2k3 * k2 ^ 2;
    mddH_i_in_im1_dk3dk3_12 = -sk1 * ck1 * ck2k3 * k2 ^ 2;
    mddH_i_in_im1_dk3dk3_13 = -ck1 * sk2k3 * k2 ^ 2;
    mddH_i_in_im1_dk3dk3_14 = ck1 * ck2k3 * k2;
    
    mddH_i_in_im1_dk3dk3_21 = -sk1 * ck1 * ck2k3 * k2 ^ 2;
    mddH_i_in_im1_dk3dk3_22 = -ck2k3 * k2 ^ 2 * sk1 ^ 2;
    mddH_i_in_im1_dk3dk3_23 = -sk1 * sk2k3 * k2 ^ 2;
    mddH_i_in_im1_dk3dk3_24 = sk1 * ck2k3 * k2;
    
    mddH_i_in_im1_dk3dk3_31 = ck1 * sk2k3 * k2 ^ 2;
    mddH_i_in_im1_dk3dk3_32 = sk1 * sk2k3 * k2 ^ 2;
    mddH_i_in_im1_dk3dk3_33 = -ck2k3 * k2 ^ 2;
    mddH_i_in_im1_dk3dk3_34 = -sk2k3 * k2;
    
    ddH_I1_I0_dk_I_dk_I(9:11, 9:12)     = [mddH_i_in_im1_dk3dk3_11, mddH_i_in_im1_dk3dk3_12, mddH_i_in_im1_dk3dk3_13, mddH_i_in_im1_dk3dk3_14;
                                           mddH_i_in_im1_dk3dk3_21, mddH_i_in_im1_dk3dk3_22, mddH_i_in_im1_dk3dk3_23, mddH_i_in_im1_dk3dk3_24;
                                           mddH_i_in_im1_dk3dk3_31, mddH_i_in_im1_dk3dk3_32, mddH_i_in_im1_dk3dk3_33, mddH_i_in_im1_dk3dk3_34 ]; 
                                       
    % d2H_i_in_im1_dk1dk2 = d2H_i_in_im1_dk2dk1
    mddH_i_in_im1_dk1dk2_11 = 0.2e1 * sk1 * ck1 * sk2k3 * k3;
    mddH_i_in_im1_dk1dk2_12 = -sk2k3 * k3 * (0.2e1 * ck1 ^ 2 - 0.1e1);
    mddH_i_in_im1_dk1dk2_13 = -sk1 * ck2k3 * k3;
    mddH_i_in_im1_dk1dk2_14 = -sk1 * (sk2k3 * k3 * k2 + ck2k3 - 0.1e1) / k2 ^ 2;
    
    mddH_i_in_im1_dk1dk2_21 = -sk2k3 * k3 * (0.2e1 * ck1 ^ 2 - 0.1e1);
    mddH_i_in_im1_dk1dk2_22 = -0.2e1 * sk1 * ck1 * sk2k3 * k3;
    mddH_i_in_im1_dk1dk2_23 = ck1 * ck2k3 * k3;
    mddH_i_in_im1_dk1dk2_24 = ck1 * (sk2k3 * k3 * k2 + ck2k3 - 0.1e1) / k2 ^ 2;
    
    mddH_i_in_im1_dk1dk2_31 = sk1 * ck2k3 * k3;
    mddH_i_in_im1_dk1dk2_32 = -ck1 * ck2k3 * k3;
    mddH_i_in_im1_dk1dk2_33 = 0;
    mddH_i_in_im1_dk1dk2_34 = 0;
    
    ddH_I1_I0_dk_I_dk_I(1:3, 5:8)       = [mddH_i_in_im1_dk1dk2_11, mddH_i_in_im1_dk1dk2_12, mddH_i_in_im1_dk1dk2_13, mddH_i_in_im1_dk1dk2_14;
                                           mddH_i_in_im1_dk1dk2_21, mddH_i_in_im1_dk1dk2_22, mddH_i_in_im1_dk1dk2_23, mddH_i_in_im1_dk1dk2_24;
                                           mddH_i_in_im1_dk1dk2_31, mddH_i_in_im1_dk1dk2_32, mddH_i_in_im1_dk1dk2_33, mddH_i_in_im1_dk1dk2_34 ]; 
    ddH_I1_I0_dk_I_dk_I(5:7, 1:4) = ddH_I1_I0_dk_I_dk_I(1:3, 5:8);
    
    % d2H_i_in_im1_dk1dk3 = d2H_i_in_im1_dk3dk1
    mddH_i_in_im1_dk1dk3_11 = 0.2e1 * sk1 * ck1 * sk2k3 * k2;
    mddH_i_in_im1_dk1dk3_12 = -sk2k3 * k2 * (0.2e1 * ck1 ^ 2 - 0.1e1);
    mddH_i_in_im1_dk1dk3_13 = -sk1 * ck2k3 * k2;
    mddH_i_in_im1_dk1dk3_14 = -sk1 * sk2k3;
    
    mddH_i_in_im1_dk1dk3_21 = -sk2k3 * k2 * (0.2e1 * ck1 ^ 2 - 0.1e1);
    mddH_i_in_im1_dk1dk3_22 = -0.2e1 * sk1 * ck1 * sk2k3 * k2;
    mddH_i_in_im1_dk1dk3_23 = ck1 * ck2k3 * k2;
    mddH_i_in_im1_dk1dk3_24 = ck1 * sk2k3;
    
    mddH_i_in_im1_dk1dk3_31 = sk1 * ck2k3 * k2;
    mddH_i_in_im1_dk1dk3_32 = -ck1 * ck2k3 * k2;
    mddH_i_in_im1_dk1dk3_33 = 0;
    mddH_i_in_im1_dk1dk3_34 = 0;
    
    ddH_I1_I0_dk_I_dk_I(1:3, 9:12)      = [mddH_i_in_im1_dk1dk3_11, mddH_i_in_im1_dk1dk3_12, mddH_i_in_im1_dk1dk3_13, mddH_i_in_im1_dk1dk3_14;
                                           mddH_i_in_im1_dk1dk3_21, mddH_i_in_im1_dk1dk3_22, mddH_i_in_im1_dk1dk3_23, mddH_i_in_im1_dk1dk3_24;
                                           mddH_i_in_im1_dk1dk3_31, mddH_i_in_im1_dk1dk3_32, mddH_i_in_im1_dk1dk3_33, mddH_i_in_im1_dk1dk3_34 ]; 
    ddH_I1_I0_dk_I_dk_I(9:11, 1:4) = ddH_I1_I0_dk_I_dk_I(1:3, 9:12);
    
    % d2H_i_in_im1_dk2dk3 = d2H_i_in_im1_dk3dk2
    mddH_i_in_im1_dk2dk3_11 = -ck1 ^ 2 * (ck2k3 * k3 * k2 + sk2k3);
    mddH_i_in_im1_dk2dk3_12 = -sk1 * ck1 * (ck2k3 * k3 * k2 + sk2k3);
    mddH_i_in_im1_dk2dk3_13 = ck1 * (-sk2k3 * k3 * k2 + ck2k3);
    mddH_i_in_im1_dk2dk3_14 = ck1 * ck2k3 * k3;
    
    mddH_i_in_im1_dk2dk3_21 = -sk1 * ck1 * (ck2k3 * k3 * k2 + sk2k3);
    mddH_i_in_im1_dk2dk3_22 = -sk1 ^ 2 * (ck2k3 * k3 * k2 + sk2k3);
    mddH_i_in_im1_dk2dk3_23 = sk1 * (-sk2k3 * k3 * k2 + ck2k3);
    mddH_i_in_im1_dk2dk3_24 = sk1 * ck2k3 * k3;
    
    mddH_i_in_im1_dk2dk3_31 = -ck1 * (-sk2k3 * k3 * k2 + ck2k3);
    mddH_i_in_im1_dk2dk3_32 = -sk1 * (-sk2k3 * k3 * k2 + ck2k3);
    mddH_i_in_im1_dk2dk3_33 = -ck2k3 * k3 * k2 - sk2k3;
    mddH_i_in_im1_dk2dk3_34 = -sk2k3 * k3;
    
    ddH_I1_I0_dk_I_dk_I(5:7, 9:12)      = [mddH_i_in_im1_dk2dk3_11, mddH_i_in_im1_dk2dk3_12, mddH_i_in_im1_dk2dk3_13, mddH_i_in_im1_dk2dk3_14;
                                           mddH_i_in_im1_dk2dk3_21, mddH_i_in_im1_dk2dk3_22, mddH_i_in_im1_dk2dk3_23, mddH_i_in_im1_dk2dk3_24;
                                           mddH_i_in_im1_dk2dk3_31, mddH_i_in_im1_dk2dk3_32, mddH_i_in_im1_dk2dk3_33, mddH_i_in_im1_dk2dk3_34 ]; 
    ddH_I1_I0_dk_I_dk_I(9:11, 5:8) = ddH_I1_I0_dk_I_dk_I(5:7, 9:12);
end

% HHHHHHHHHHHHH Partielle Ableitung der Zeitableitung von H HHHHHHHHHHHHHHHHHHHHHHHH
function [H_2_in_0] = clc_Trafo_H(H_1_in_0, H_2_in_1)
% Input:
%   - Eine Matrix [4x4]
%   - Eine Matrix [4*nz x 4*ns]
%
% Output:
%   - H_2_in_0 [4*n x 4*ns] = H_1_in_0*H_2_in_1

    [nz1, ns1] = size(H_1_in_0);
    [nz2, ns2] = size(H_2_in_1);

    nz_max = max(nz1./4, nz2./4);
    ns_max = max(ns1./4, ns2./4);

    H_2_in_0 = zeros(4*nz_max, 4*ns_max);

    if (nz1+ns1) < (nz2+ns2)
        for zz = 1:nz_max
            for ss = 1:ns_max
                H_2_in_0((1:4)+4*(zz-1), (1:4)+4*(ss-1)) = H_1_in_0 * H_2_in_1((1:4)+4*(zz-1), (1:4)+4*(ss-1));
            end
        end
    else
        for zz = 1:nz_max
            for ss = 1:ns_max
                H_2_in_0((1:4)+4*(zz-1), (1:4)+4*(ss-1)) = H_1_in_0((1:4)+4*(zz-1), (1:4)+4*(ss-1)) * H_2_in_1;
            end
        end
    end
end

== matlab function libbha_kinematic/BHA_Kin_NumDiff_1stO_CC_cont/createForMatrix ==
  data: q input size=[9,1]; q_plus_dq output size=[9,1,9]; dq input size=[9,1]; q_minus_dq output size=[9,1,9]; norm_dq output size=[1,1,9]
function [q_plus_dq, q_minus_dq, norm_dq] = createForMatrix(q, dq)
% Input:
% q     [nx1]   Zustand Gelenkvariablen
% dq    [nx1]   Betrag der differentiellen Aenderung je Gelenkzustand zur
%               Ableitungsbestimmung (->Jacobimatrix)
%
% Output:
% qpdq  [nx1xn] Gelenkzustand zuzüglich diferentieller Änderung
%               Reihenfolge: nx1x1 = [q1+dq1; q2; ...; qn]
%                            nx1x2 = [q1; q2+dq2; ...; qn] 
%                                  : 
%                            nx1xn = [q1; q2; ...; qn+dqn]
% qmdq  [nx1xn] Gelenkzustand abzüglich diferentieller Änderung
%               Reihenfolge: nx1x1 = [q1-dq1; q2; ...; qn]
%                            nx1x2 = [q1; q2-dq2; ...; qn] 
%                                  : 
%                            nx1xn = [q1; q2; ...; qn-dqn] 
% ndq   [1x1xn] Norm der differentiellen Änderung

n               = 9;
q_plus_dq       = zeros(n,1,n);
q_minus_dq      = zeros(n,1,n);
norm_dq         = zeros(1,1,n);

dq_vec          = reshape(diag(dq),n,1,n);
norm_dq(1,1,:)  = dq;

for ii = 1:n
    q_plus_dq(:,:,ii)   =q+dq_vec(:,:,ii);
    q_minus_dq(:,:,ii)  =q-dq_vec(:,:,ii);
end

== matlab function libbha_kinematic/BHA_Kin_Dir_ExtFixedTool ==
  data: H_tool input; h_toolbase input; h output
function h    = Jacobi_CC_continuum(H_tool, h_toolbase)
% XXXXXXXXXXXXXXXXXXXXXXXXXXXXXXXXXXXXXXXXXXXXXXXXXXXXXXXXXXXXXXXXXXXXXXXXX
% Analytische Berechnung der Jacobi-Matrix J_general bei Verwendung einer
% zusätzlichen konstanten Handachse
% - Modell - Constant Curvature Continuum
%
% Ansatz:
% h = h_general ** H                    ** ist hierbei die Matrizenmultiplikation der homogenen Matrizen. h muss zuvor in H konvertiert werden
% J_general_toolbase = J_general ** H
%
% mit:
% h     = [ H_1,1,  H_2,1,  H_3,1,  H_1,2,  H_2,2,  H_3,2,  H_1,3,  H_2,3,  H_3,3,  H_1,4,  H_2,4,  H_3,4]
%           1       2       3       4       5       6       7       8       9       10      11      12   
%
% Input:
%   H_tool               [4x4]   Homogene Transformation: Koordinatensystem TCP
%                                relativ zum Werkzeugansatz
%   h_toolbase           [12x1]  Pose des Werkzeugansatzes (Homogene Transformation in Vektor geschrieben, ohne Zeile 0,0,0,1)
%   J_allg_toolbase      [12x3n] Jacobi-Matrix des Werkzeugansatzes
%
% Output:
%   h                    [12x1]  Pose des TCP (Homogene Transformation in Vektor geschrieben, ohne Zeile 0,0,0,1)
%   J_allg               [12x3n] Allgemeingültige Jacobi-Matrix für kontinuierliche Manipulatoren
%
% Parameter:
%   n                    [1x1]   Anzahl der Sektionen
%
% Stand: 10.04.2013      Valentin Falkenhahn
% XXXXXXXXXXXXXXXXXXXXXXXXXXXXXXXXXXXXXXXXXXXXXXXXXXXXXXXXXXXXXXXXXXXXXXXXX
    
    h = htH(h_toolbase,H_tool);
end

% XXXXXXXXXXXXXXXXXXXXXXXXXXXXXXX HELPER XXXXXXXXXXXXXXXXXXXXXXXXXXXXXXXXX

function res = htH(h1,H)
    res = H2h(h2H(h1)*H);
end

function H = h2H(h)
    H= [[h(1:3), h(4:6), h(7:9), h(10:12)]; [0 0 0 1]];
end

function h = H2h(H)
         h = [H(1:3,1);
         H(1:3,2);
         H(1:3,3);
         H(1:3,4)];
end
